simulink model "schemat_osc"  (R2020a)
settings: Solver=VariableStepAuto  StartTime=0.0  StopTime=10.0  MaxStep=0.01  RelTol=1e-3
values from neighbouring files (symbols this model uses):
  a = 0    [lab5ok.m]
  du = 1    [lab5ok.m]
  ksi = [0.9, 0.4, 0.9, 0.4]    [lab5ok.m]
  u0 = 0    [lab5ok.m]
  wn = [(2/0.9), 1, 1, 5]    [lab5ok.m]
  x0 = 0    [lab5ok.m]
  x10 = 0    [lab5ok.m]
settings Model: Creator=pc  LastModifiedBy=pc

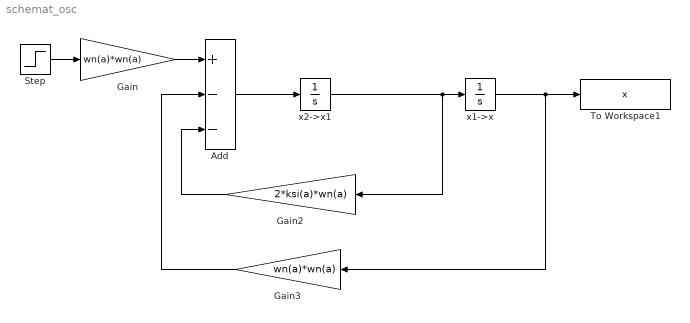
== system schemat_osc ==
  Add : Sum  Inputs=+--
  Gain : Gain  Gain=wn(a)*wn(a)
  Gain2 : Gain  Gain=2*ksi(a)*wn(a)
  Gain3 : Gain  Gain=wn(a)*wn(a)
  Step : Step  Time=2  Before=u0  After=u0+du  SampleTime=1
  To Workspace1 : ToWorkspace  VariableName=x  SampleTime=-1
  x1->x : Integrator  InitialCondition=x0
  x2->x1 : Integrator  InitialCondition=x10
  wires:
  Gain2/1 -> Add/3
  x2->x1/1 -> x1->x/1, Gain2/1
  Gain3/1 -> Add/2
  x1->x/1 -> To Workspace1/1, Gain3/1
  Step/1 -> Gain/1
  Add/1 -> x2->x1/1
  Gain/1 -> Add/1
